simulink model "demux"  (Simulink 7.6)
settings: Solver=FixedStepDiscrete  StartTime=0.0  StopTime=10.0  FixedStep=1  RelTol=1e-3
settings Model: Creator=ksmyth  LastModifiedBy=hnine
settings OptimizationCC: InitFltsAndDblsToZero=on
settings DebuggingCC: SaveWithParameterizedLinksMsg=none  StrictBusMsg=Warning
settings GRTTargetCC: TargetFcnLib=ansi_tfl_tmw.mat

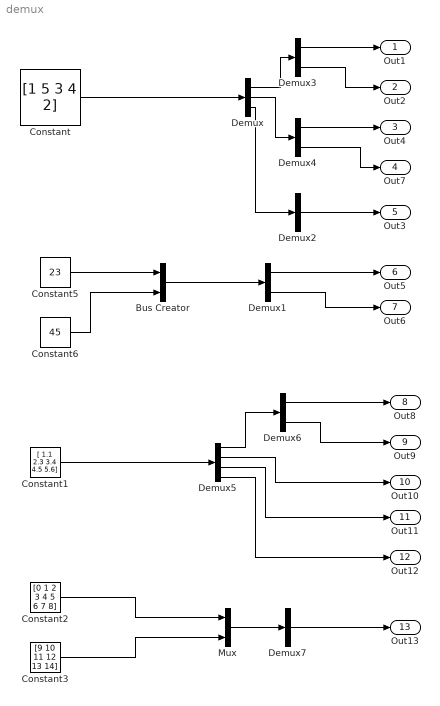
== system demux ==
  Bus Creator : BusCreator  Inputs=2
  Constant : Constant  Value=[1 5 3 4 2]
  Constant1 : Constant  Value=[ 1.1 2.3 3.4 4.5 5.6]
  Constant2 : Constant  Value=[0 1 2 3 4 5 6 7 8]
  Constant3 : Constant  Value=[9 10 11 12 13 14]
  Constant5 : Constant  Value=23
  Constant6 : Constant  Value=45
  Demux : Demux  Outputs=3
  Demux1 : Demux  Outputs=2  BusSelectionMode=on
  Demux2 : Demux  Outputs=1
  Demux3 : Demux  Outputs=2
  Demux4 : Demux  Outputs=2
  Demux5 : Demux
  Demux6 : Demux  Outputs=2
  Demux7 : Demux  Outputs=1
  Mux : Mux  Inputs=2
  Out1 : Outport
  Out2 : Outport  Port=2
  Out4 : Outport  Port=3
  Out7 : Outport  Port=4
  Out3 : Outport  Port=5
  Out5 : Outport  Port=6
  Out6 : Outport  Port=7
  Out8 : Outport  Port=8
  Out9 : Outport  Port=9
  Out10 : Outport  Port=10
  Out11 : Outport  Port=11
  Out12 : Outport  Port=12
  Out13 : Outport  Port=13
  wires:
  Constant5/1 -> Bus Creator/1
  Bus Creator/1 -> Demux1/1
  Constant6/1 -> Bus Creator/2
  Constant/1 -> Demux/1
  Demux/3 -> Demux2/1
  Demux2/1 -> Out3/1
  Demux1/1 -> Out5/1
  Demux1/2 -> Out6/1
  Demux/2 -> Demux4/1
  Demux/1 -> Demux3/1
  Demux3/1 -> Out1/1
  Demux3/2 -> Out2/1
  Demux4/1 -> Out4/1
  Demux4/2 -> Out7/1
  Constant1/1 -> Demux5/1
  Demux5/1 -> Demux6/1
  Demux6/1 -> Out8/1
  Demux6/2 -> Out9/1
  Demux5/2 -> Out10/1
  Demux5/3 -> Out11/1
  Demux5/4 -> Out12/1
  Mux/1 -> Demux7/1
  Demux7/1 -> Out13/1
  Constant2/1 -> Mux/1
  Constant3/1 -> Mux/2
